simulink library "SignalPreprocessingLib"  (R2020b)
settings: Solver=VariableStepAuto  StartTime=0.0  StopTime=10.0  RelTol=1e-3
undefined symbols (not defined in the file or in its folder): fdesignblkfcn, fs, gcbh, param_ecg_gain_mv
(part 3 of 7)

== system SignalPreprocessingLib/FiltFilter/Enabled Filtfiltering Subsystem/Filtfiltering/Bandpass Filter 1 ==
  In : Inport
  Generated Filter Block : DiscreteFir  Tag=BlockMethodSubSystem  Coefficients=[-0.0114243088354877773 0.00587624110456374388 0.00413946068324517157 0.00264334557424035672 0.00138774422276622192 0.00039597756815762733 -0.000357391963790950132 -0.000870027328167087902 -0.00118474210009046274 -0.0013114772414377189 -0.00130211118137258525 -0.00117028348293094116 -0.000969555288066135598 -0.000709991739662891794 -0.000441672338585462343 -0.000165596169411169614 7.38618239838010476e-05 0.000289182992126718261 0.00043918297873611449 0.000554539538172022298 0.000596791094711021305 0.000591852861038305242 0.000558642096174625374 0.000449318410474004379 0.000334719809825502479 0.00020575650819831294 5.39363215079843861e-05 -0.000101322531501510382 -0.000240833690149395291 -0.000354646039305753225 -0.000451018706232981029 -0.000523127741752206499 -0.000570171746042747937 -0.000579976289078059509 -0.000560050610609794802 -0.000510203484091005868 -0.000444253999700439106 -0.000361620699264023418 -0.000270418439597897714 -0.000171285996548194847 -6.96491449474114649e-05 2.51074882581126674e-05 0.000107701466472475207 0.000177443554931332875 0.000215288445749358542 0.000245848468855064048 0.000245696970898627229 0.000229649686627229205 0.00019096241212286473 0.000142984412950488554 7.04459950623022302e-05 -8.24128026295257998e-06 -9.80593727097200246e-05 -0.000181512369773678683 -0.000268731962362029828 -0.000342263684306691809 -0.000409113387221587271 -0.000453067377901137172 -0.000486836085121275519 -0.000497275928952340546 -0.00049828288783324709 -0.000472232231767717378 -0.00043821960462679492 -0.000378588991066479766 -0.000316844305738618603 -0.000241178452312015845 -0.000166037327502541535 -8.72939132895780845e-05 -1.92312446675550752e-05 4.72061762121969014e-05 9.32922079647201252e-05 0.000128677828260322091 0.000142225646220916352 0.000145392718308013161 0.000124316294889322346 9.22525950362868691e-05 3.91139366419743922e-05 -2.09540055264127723e-05 -9.84817072707550728e-05 -0.000176447200533612 -0.000261969930569216219 -0.000338398170707415388 -0.000413673787246831778 -0.000474956484152477126 -0.000526126847064748229 -0.000557031780194342657 -0.000573463759814568652 -0.000565518328802135789 -0.000545968260267525388 -0.000503292825521842527 -0.000450686144492560767 -0.00038193732270500047 -0.000310533512604118864 -0.000229221000311531989 -0.000153634622944792687 -7.7008709436998668e-05 -1.29951882972875049e-05 4.41972427699440645e-05 7.97744827227258452e-05 0.000101355022460052069 9.88614688825825011e-05 8.13696224336354218e-05 3.98982051577762009e-05 -1.42484593806998378e-05 -8.82654671942838254e-05 -0.000167074457359766074 -0.00025963077237387 -0.000347989994374806391 -0.000439444994547399936 -0.00051811479354047299 -0.000590082617058047473 -0.000641838802120880611 -0.000681503522967578934 -0.000694804478821137508 -0.00069209853970065606 -0.000663795693677639645 -0.000621757222242421206 -0.000557224399686986893 -0.000484587241980041772 -0.000396687438130890677 -0.000308737174406251494 -0.000214743893139471981 -0.00013218336614707546 -5.38482479860227792e-05 3.99111044497961476e-06 4.92154210607297082e-05 6.74354760492514721e-05 6.74472479585495194e-05 4.02217001782036176e-05 -4.06942016077313506e-06 -7.33562872444193381e-05 -0.000154074998390272069 -0.000252782754343081062 -0.000354062465090758047 -0.000462222943123069205 -0.000562271536985421011 -0.000658661832374597689 -0.000735808311790427799 -0.000799943578584080828 -0.000838241882526128551 -0.000857844739487072239 -0.000847533102258754556 -0.000817418121589637975 -0.000760200301916437102 -0.000687422833072246636 -0.000595027809558780832 -0.000496080524377292761 -0.000387710990138089018 -0.000284208196984854847 -0.000182518571703508756 -9.84384035011120345e-05 -2.73607674165961268e-05 1.77508990696524649e-05 4.21653277528823839e-05 3.53040248291924125e-05 5.59921773045889137e-06 -5.46825757556310132e-05 -0.000133739024050423885 -0.000236066993422962002 -0.000348549704079315764 -0.000473403235651745358 -0.000595572390038458938 -0.000716976323207035166 ...(+20655 chars)]  InputProcessing=Columns as channels (frame based)
  Out : Outport  VectorParamsAs1DForOutWhenUnconnected=off
  wires:
  In/1 -> Generated Filter Block/1
  Generated Filter Block/1 -> Out/1
